simulink model "model"  (R2020b)
settings: Solver=VariableStepAuto  StartTime=0.0  StopTime=10.0  RelTol=1e-3
settings Model: Creator=rishavgoenka  LastModifiedBy=rishavgoenka

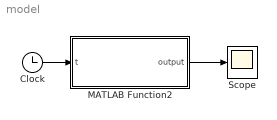
== system model ==
  Clock : Clock
  MATLAB Function2 : MATLAB Function  TreatAsAtomicUnit=on
  Scope : Scope
  wires:
  Clock/1 -> MATLAB Function2/1(t)
  MATLAB Function2/1(output) -> Scope/1

== matlab function model/MATLAB Function2 ==
  data: output output; t input
function output = generate_circle(t)
output = [cos(t), sin(t)];
end
